simulink model "Dyn_PointMass_R2015B"  (R2015b)
settings: Solver=ode4  SolverMode=SingleTasking  StartTime=0.0  StopTime=simInit.TSIM  FixedStep=simInit.dt  MaxStep=simInit.dt  RelTol=1e-3
InitFcn:
  | close all
undefined symbols (not defined in the file): base_windspeed, constr, DE2019, DiscIntNeverNeededParam, ENVMT, Lbooth, loiterStates, params, simInit, T, winchParameter
libraries: simulink x40, simulink_extras x3, dspsigops x1
(part 4 of 5)

== matlab function Dyn_PointMass_R2015B/AirborneSystem/AeroAndPropForces/Aero_prop ==
  data: F_p_B output; airdata input; DE2019 parameter; delta_t input; F_a_B output; cl_w input; cd_w input; cl_e input; cd_e input; cl_r input; cd_r input; ENVMT parameter
% Copyright 2020 Delft University of Technology
%
% Licensed under the Apache License, Version 2.0 (the "License");
% you may not use this file except in compliance with the License.
% You may obtain a copy of the License at
%
%      http://www.apache.org/licenses/LICENSE-2.0
%
% Unless required by applicable law or agreed to in writing, software
% distributed under the License is distributed on an "AS IS" BASIS,
% WITHOUT WARRANTIES OR CONDITIONS OF ANY KIND, either express or implied.
% See the License for the specific language governing permissions and
% limitations under the License.

function [F_p_B,F_a_B] = simpleAero(airdata, DE2019, delta_t,cl_w,cd_w,cl_e,cd_e,cl_r,cd_r, ENVMT)
%simpleAero - Calculate aerodynamic and propulsive forces
%
% Syntax:  [F_p_B,F_a_B] = simpleAero(airdata, aircraft_struct, delta_t,cl_w,cd_w,cl_e,cd_e,cl_r,cd_r)
%
% Inputs:
%    airdata - Wind speed, angle of attack and side slip angle
%    DE2019 - Aircraft characteristics data structure
%    delta_t - Thrust force
%    cl_w - Lift coefficient wing
%    cd_w - Drag coefficient wing
%    cl_e - Lift coefficient elevator
%    cd_e - Drag coefficient elevator
%    cl_r - Lift coefficient rudder
%    cd_r - Drag coefficient rudder
%
% Outputs:
%    F_p_B  - Propulsive forces in body reference frame
%    F_a_B  - Total aircraft aerodynamic forces in body reference frame
%   
% Example: 
%    [F_p_B,F_a_B] = simpleAero(airdata, DE2019, delta_t,cl_w,cd_w,cl_e,cd_e,cl_r,cd_r)
%
% Other m-files required: none
% Subfunctions: none
% MAT-files required: none
%
% Author: Dylan Eijkelhof, M.Sc.
% Delft University of Technology
% email address: d.eijkelhof@tudelft.nl  
% December 2019; Last revision: 30-September-2019

%------------- BEGIN CODE --------------    
    F_a_B = zeros(3,1);
    F_p_B = zeros(3,1);

    Va = airdata(1);
    alpha = airdata(2);
    beta = airdata(3);    
    Vinf = [Va*cos(alpha)*cos(beta), Va*sin(beta), Va*sin(alpha)*cos(beta)];

    q = 0.5*ENVMT.rhos*Vinf(1)^2;
    
    %% Main Wing
    F_L_main = -cl_w*q*DE2019.S_ref;
    F_D_main = cd_w*q*DE2019.S_ref;
    
    F_x_mw = -F_D_main*cos(alpha) - F_L_main*sin(alpha);
    F_z_mw = F_L_main*cos(alpha);

    %% Elevator
    F_L_el = -cl_e*q*DE2019.S_el;
    F_D_el = -cd_e*q*DE2019.S_el;
    
    F_x_el = F_D_el*cos(alpha)*cos(beta) - F_L_el*sin(alpha)*cos(beta);
    F_z_el = F_L_el*cos(alpha);
   
    %% Rudder
    F_L_vs = 2*cl_r*q*DE2019.S_vs;
    F_D_vs = -2*cd_r*q*DE2019.S_vs;

    F_x_vs = F_D_vs*cos(alpha)*cos(beta);
    F_y_vs = -F_L_vs*cos(beta);
    
    %% Sum of forces
    F_a_B = [F_x_mw+F_x_el+F_x_vs;F_y_vs; F_z_mw+F_z_el];
    
    %% Motor
%     Vd = airdata(1) + delta_t * ( DE2019.k_motor - airdata(1) );
%     Fp_x = 0.5 * 1.225 * DE2019.S_prop * DE2019.C_prop * Vd * (Vd-airdata(1));
    %% No motor, direct feed through
    F_p_B = [delta_t;0;0];
%------------- END CODE -------------- 
end
%

== matlab function Dyn_PointMass_R2015B/AirborneSystem/FlightControlSystem/AirspeedController_SS_1/Airspeed_Brake/FeedforwardPart ==
  data: gamma input; BF output; nu_V input; ENVMT parameter; Drag_force input; DE2019 parameter
% Copyright 2021 Delft University of Technology
%
% Licensed under the Apache License, Version 2.0 (the "License");
% you may not use this file except in compliance with the License.
% You may obtain a copy of the License at
%
%      http://www.apache.org/licenses/LICENSE-2.0
%
% Unless required by applicable law or agreed to in writing, software
% distributed under the License is distributed on an "AS IS" BASIS,
% WITHOUT WARRANTIES OR CONDITIONS OF ANY KIND, either express or implied.
% See the License for the specific language governing permissions and
% limitations under the License.

function BF = feedforward_brake(gamma, nu_V,  ENVMT, Drag_force, DE2019)
%feedforward_brake - Brake force calculation for velocity decrease
%
% Inputs:
%    gamma      - Path angle (glideslope)
%    nu_V       - Controlled velocity parameter
%    ENVMT      - Environmental characteristics
%    Drag_force	- Drag
%    DE2019     - Aircraft characteristics
%
% Outputs:
%    BF          - Brake force
%
% Example: 
%    BF = feedforward_thrust(gamma, nu_V,  ENVMT, Drag_force, DE2019)
%
% Author: Sebastian Rapp, Ph.D., Revised by: Dylan Eijkelhof, M.Sc.
% Delft University of Technology
% email address: s.rapp@tudelft.nl
% email address: d.eijkelhof@tudelft.nl
% December 2019; Last revision: 06-October-2020

%-------------	BEGIN CODE	--------------

BF = DE2019.mass * ( ENVMT.g * sin(gamma) + nu_V ) + Drag_force; % required thrust

%-------------	 END CODE	--------------
end

== matlab function Dyn_PointMass_R2015B/AirborneSystem/FlightControlSystem/AirspeedController_SS_1/Airspeed_Brake/MATLAB Function ==
  data: F_a_B input; Drag output; AoA input
% Copyright 2021 Delft University of Technology
%
% Licensed under the Apache License, Version 2.0 (the "License");
% you may not use this file except in compliance with the License.
% You may obtain a copy of the License at
%
%      http://www.apache.org/licenses/LICENSE-2.0
%
% Unless required by applicable law or agreed to in writing, software
% distributed under the License is distributed on an "AS IS" BASIS,
% WITHOUT WARRANTIES OR CONDITIONS OF ANY KIND, either express or implied.
% See the License for the specific language governing permissions and
% limitations under the License.

function Drag  = estimate_drag(F_a_B, AoA)
%estimate_drag - Transform drag from B to A reference frame
%
% Inputs:
%    F_a_B     - Aerodynamic forces in body reference frame
%    AoA       - Angle of Attack
%
% Outputs:
%    Drag    - Drag force
%
% Example: 
%    [Drag] = estimate_drag(F_a_B, AoA)
%
% Author: Sebastian Rapp, Ph.D., Revised by: Dylan Eijkelhof, M.Sc.
% Delft University of Technology
% email address: s.rapp@tudelft.nl
% email address: d.eijkelhof@tudelft.nl
% December 2019; Last revision: 06-October-2020

%-------------	BEGIN CODE	--------------

F_a_A = [cos(AoA), 0, sin(AoA);
    0, 1, 0; 
    -sin(AoA), 0, cos(AoA)] * F_a_B;

Drag = -F_a_A(1);

%-------------	 END CODE	--------------

end

== matlab function Dyn_PointMass_R2015B/AirborneSystem/FlightControlSystem/AirspeedController_SS_1/Airspeed_Brake/hedging ==
  data: Drag_force input; gamma input; nu_V output; BF input; ENVMT parameter; DE2019 parameter
% Copyright 2021 Delft University of Technology
%
% Licensed under the Apache License, Version 2.0 (the "License");
% you may not use this file except in compliance with the License.
% You may obtain a copy of the License at
%
%      http://www.apache.org/licenses/LICENSE-2.0
%
% Unless required by applicable law or agreed to in writing, software
% distributed under the License is distributed on an "AS IS" BASIS,
% WITHOUT WARRANTIES OR CONDITIONS OF ANY KIND, either express or implied.
% See the License for the specific language governing permissions and
% limitations under the License.

function nu_V = hedgingV(Drag_force, gamma, BF, ENVMT, DE2019)

%hedgingV
%
% Inputs:
%    Drag_force	- Drag
%    gamma      - Path angle (glideslope)
%    BF         - Brake force
%    ENVMT      - Environmental characteristics
%    DE2019     - Aircraft characteristics
%
% Outputs:
%    nu_V       - Controlled velocity parameter
%
% Example: 
%    nu_V = hedgingV(Drag_force, gamma, BF, ENVMT, DE2019)
%
% Author: Sebastian Rapp, Ph.D., Revised by: Dylan Eijkelhof, M.Sc.
% Delft University of Technology
% email address: s.rapp@tudelft.nl
% email address: d.eijkelhof@tudelft.nl
% December 2019; Last revision: 06-October-2020

%-------------	BEGIN CODE	--------------

nu_V = (BF-Drag_force)/DE2019.mass - ENVMT.g * sin(gamma); 

%-------------	 END CODE	--------------
end

== matlab function Dyn_PointMass_R2015B/RequirementModelsAndLogging/MATLAB Function ==
  data: time input; eul input; stop_flag output; eul_old input
% Copyright 2021 Delft University of Technology
%
% Licensed under the Apache License, Version 2.0 (the "License");
% you may not use this file except in compliance with the License.
% You may obtain a copy of the License at
%
%      http://www.apache.org/licenses/LICENSE-2.0
%
% Unless required by applicable law or agreed to in writing, software
% distributed under the License is distributed on an "AS IS" BASIS,
% WITHOUT WARRANTIES OR CONDITIONS OF ANY KIND, either express or implied.
% See the License for the specific language governing permissions and
% limitations under the License.

function stop_flag = fcn(time, eul,eul_old)
phi = eul(1);
theta = eul(2);
% psi = eul(3);

phi_old = eul_old(1);
theta_old = eul_old(2);
% psi_old = eul_old(3);

if time>40
    if ((phi>pi/2 || phi<-pi/2) && sign(phi) ~= sign(phi_old))
        stop_flag = 1;
    elseif ((theta>pi/2 || theta<-pi/2) && sign(theta) ~= sign(theta_old))
        stop_flag = 1; 
%     elseif ((psi>pi/2 || psi<-pi/2) && sign(psi) ~= sign(psi_old))
%         stop_flag = 1; 
    else
        stop_flag = 0;
    end
else
    stop_flag = 0;
end
end

== matlab function Dyn_PointMass_R2015B/RequirementModelsAndLogging/MATLAB Function1 ==
  data: Lift output; F_a_B input; Drag output; AoA input
% Copyright 2021 Delft University of Technology
%
% Licensed under the Apache License, Version 2.0 (the "License");
% you may not use this file except in compliance with the License.
% You may obtain a copy of the License at
%
%      http://www.apache.org/licenses/LICENSE-2.0
%
% Unless required by applicable law or agreed to in writing, software
% distributed under the License is distributed on an "AS IS" BASIS,
% WITHOUT WARRANTIES OR CONDITIONS OF ANY KIND, either express or implied.
% See the License for the specific language governing permissions and
% limitations under the License.

function [Lift, Drag]  = estimate_drag(F_a_B, AoA)
%estimate_drag - Transform drag from B to A reference frame
%
% Inputs:
%    F_a_B     - Aerodynamic forces in body reference frame
%    AoA       - Angle of Attack
%
% Outputs:
%    Drag    - Drag force
%
% Example: 
%    [Drag] = estimate_drag(F_a_B, AoA)
%
% Author: Sebastian Rapp, Ph.D., Revised by: Dylan Eijkelhof, M.Sc.
% Delft University of Technology
% email address: s.rapp@tudelft.nl
% email address: d.eijkelhof@tudelft.nl
% December 2019; Last revision: 06-October-2020

%-------------	BEGIN CODE	--------------

F_a_A = [cos(AoA), 0, sin(AoA);
    0, 1, 0; 
    -sin(AoA), 0, cos(AoA)] * F_a_B;

Lift = -F_a_A(3);
Drag = -F_a_A(1);

%-------------	 END CODE	--------------

end

== matlab function Dyn_PointMass_R2015B/AirborneSystem/FlightControlSystem/PathFollowingController_SS_2/FlightOnFlatEarth (Retraction&Loitering)/CalculateAttitudeCmds/FlightPathLoopRetraction_Aerodynamic/FlightpathReferenceModels/SecondOrderReferenceModel_course/wrapto2pi ==
  data: u input; y output
% Copyright 2021 Delft University of Technology
%
% Licensed under the Apache License, Version 2.0 (the "License");
% you may not use this file except in compliance with the License.
% You may obtain a copy of the License at
%
%      http://www.apache.org/licenses/LICENSE-2.0
%
% Unless required by applicable law or agreed to in writing, software
% distributed under the License is distributed on an "AS IS" BASIS,
% WITHOUT WARRANTIES OR CONDITIONS OF ANY KIND, either express or implied.
% See the License for the specific language governing permissions and
% limitations under the License.

function y = wrap_to_2pi(u)
u = mod(u, 2*pi); 
if u > pi 
    du = mod(u,pi);
    y = -pi+du; 
elseif u < -pi 
    du = mod(u,-pi); 
    y = pi+du;
else
    y = u; 
end
end

== matlab function Dyn_PointMass_R2015B/Environment_SS_3/MATLAB Function1 ==
  data: v_w_u input; v_w_p_mat output
% Copyright 2021 Delft University of Technology
%
% Licensed under the Apache License, Version 2.0 (the "License");
% you may not use this file except in compliance with the License.
% You may obtain a copy of the License at
%
%      http://www.apache.org/licenses/LICENSE-2.0
%
% Unless required by applicable law or agreed to in writing, software
% distributed under the License is distributed on an "AS IS" BASIS,
% WITHOUT WARRANTIES OR CONDITIONS OF ANY KIND, either express or implied.
% See the License for the specific language governing permissions and
% limitations under the License.

function v_w_p_mat = fcn(v_w_u)

v_w_p_mat = zeros( 3, length( v_w_u) );
v_w_p_mat(1,:) = v_w_u';

== matlab function Dyn_PointMass_R2015B/AirborneSystem/FlightControlSystem/AirspeedController_SS_1/Airspeed_Control/FeedforwardPart ==
  data: gamma input; T output; nu_V input; ENVMT parameter; Drag_force input; DE2019 parameter
% Copyright 2021 Delft University of Technology
%
% Licensed under the Apache License, Version 2.0 (the "License");
% you may not use this file except in compliance with the License.
% You may obtain a copy of the License at
%
%      http://www.apache.org/licenses/LICENSE-2.0
%
% Unless required by applicable law or agreed to in writing, software
% distributed under the License is distributed on an "AS IS" BASIS,
% WITHOUT WARRANTIES OR CONDITIONS OF ANY KIND, either express or implied.
% See the License for the specific language governing permissions and
% limitations under the License.

function T = feedforward_thrust(gamma, nu_V,  ENVMT, Drag_force, DE2019)
%feedforward_thrust - Thrust calculation for velocity initialisation
%
% Inputs:
%    gamma      - Path angle (glideslope)
%    nu_V       - Controlled velocity parameter
%    ENVMT      - Environmental characteristics
%    Drag_force	- Drag
%    DE2019     - Aircraft characteristics
%
% Outputs:
%    T          - Thrust force
%
% Example: 
%    T = feedforward_thrust(gamma, nu_V,  ENVMT, Drag_force, DE2019)
%
% Author: Sebastian Rapp, Ph.D., Revised by: Dylan Eijkelhof, M.Sc.
% Delft University of Technology
% email address: s.rapp@tudelft.nl
% email address: d.eijkelhof@tudelft.nl
% December 2019; Last revision: 06-October-2020

%-------------	BEGIN CODE	--------------

T = DE2019.mass * ( ENVMT.g * sin(gamma) + nu_V ) + Drag_force; % required thrust

% Based on the quotient of commmanded to max. available thrust
% F_T_max = ENVMT.rhos * DE2019.S_prop * DE2019.C_prop * DE2019.k_motor * (DE2019.k_motor - Va);
% delta_t = T/F_T_max; 

%-------------	 END CODE	--------------
end

== stateflow chart Dyn_PointMass_R2015B/GroundSystem_SS_4/GroundControl/Select_init_sol_for_pathfollowing ==
  state Init
    entry: sol_init = x;
  state Pumping
    entry: sol_init = transition_phi;
  (default) -> Init
  Init -> Pumping : [fm == 6]
  data: x input; fm input; sol_init output; transition_phi input

== matlab function Dyn_PointMass_R2015B/AirborneSystem/FlightControlSystem/AirspeedController_SS_1/Airspeed_Control/MATLAB Function ==
  data: F_a_B input; Drag output; AoA input
% Copyright 2021 Delft University of Technology
%
% Licensed under the Apache License, Version 2.0 (the "License");
% you may not use this file except in compliance with the License.
% You may obtain a copy of the License at
%
%      http://www.apache.org/licenses/LICENSE-2.0
%
% Unless required by applicable law or agreed to in writing, software
% distributed under the License is distributed on an "AS IS" BASIS,
% WITHOUT WARRANTIES OR CONDITIONS OF ANY KIND, either express or implied.
% See the License for the specific language governing permissions and
% limitations under the License.

function Drag = estimate_drag(F_a_B, AoA)

%estimate_drag - Transform drag from B to A reference frame
%
% Inputs:
%    F_a_B     - Aerodynamic forces in body reference frame
%    AoA       - Angle of Attack
%
% Outputs:
%    Drag    - Drag force
%
% Example: 
%    Drag = estimate_drag(F_a_B, AoA)
%
% Author: Sebastian Rapp, Ph.D., Revised by: Dylan Eijkelhof, M.Sc.
% Delft University of Technology
% email address: s.rapp@tudelft.nl
% email address: d.eijkelhof@tudelft.nl
% December 2019; Last revision: 06-October-2020

%-------------	BEGIN CODE	--------------

F_a_A = [cos(AoA), 0, sin(AoA);
    0, 1, 0; 
    -sin(AoA), 0, cos(AoA)] * F_a_B;

Drag = -F_a_A(1);

%-------------	 END CODE	--------------
end

== matlab function Dyn_PointMass_R2015B/AirborneSystem/FlightControlSystem/AirspeedController_SS_1/Airspeed_Control/hedging ==
  data: Drag_force input; gamma input; nu_V output; T input; ENVMT parameter; DE2019 parameter
% Copyright 2021 Delft University of Technology
%
% Licensed under the Apache License, Version 2.0 (the "License");
% you may not use this file except in compliance with the License.
% You may obtain a copy of the License at
%
%      http://www.apache.org/licenses/LICENSE-2.0
%
% Unless required by applicable law or agreed to in writing, software
% distributed under the License is distributed on an "AS IS" BASIS,
% WITHOUT WARRANTIES OR CONDITIONS OF ANY KIND, either express or implied.
% See the License for the specific language governing permissions and
% limitations under the License.

function nu_V = hedgingV(Drag_force, gamma, T, ENVMT, DE2019)

%hedgingV
%
% Inputs:
%    Drag_force	- Drag
%    gamma      - Path angle (glideslope)
%    T          - Thrust force
%    ENVMT      - Environmental characteristics
%    DE2019     - Aircraft characteristics
%
% Outputs:
%    nu_V       - Controlled velocity parameter
%
% Example: 
%    nu_V = hedgingV(Drag_force, gamma, T, ENVMT, DE2019)
%
% Author: Sebastian Rapp, Ph.D., Revised by: Dylan Eijkelhof, M.Sc.
% Delft University of Technology
% email address: s.rapp@tudelft.nl
% email address: d.eijkelhof@tudelft.nl
% December 2019; Last revision: 06-October-2020

%-------------	BEGIN CODE	--------------

% Based on the quotient of commmanded to max. available thrust
% F_T_max = ENVMT.rhos * DE2019.S_prop * DE2019.C_prop * DE2019.k_motor * (DE2019.k_motor - Va);
% T = F_T_max * delta_t; 

nu_V = (T-Drag_force)/DE2019.mass - ENVMT.g * sin(gamma); 

%-------------	 END CODE	--------------
end

== stateflow chart Dyn_PointMass_R2015B/AirborneSystem/FlightControlSystem/AirspeedController_SS_1/Chart ==
  state Throttle_Off
    entry: throttle_on = 0;
  state Throttle_On
    entry: throttle_on = 1;
  (default) -> Throttle_Off
  Throttle_Off -> Throttle_On : [Va<Va_min || manual_switch_on || init_throttle_flag]
  Throttle_On -> Throttle_Off : [Va>Va_min+10&&manual_switch_on==0&& init_throttle_flag ==0]
  data: Va input; Va_min input; init_throttle_flag input; throttle_on output; manual_switch_on input

== stateflow chart Dyn_PointMass_R2015B/AirborneSystem/FlightControlSystem/AirspeedController_SS_1/Chart1 ==
  state Throttle_Off
    entry: brake_on = 0;
  state Throttle_On
    entry: brake_on = 1;
  (default) -> Throttle_Off
  Throttle_Off -> Throttle_On : [(manual_switch_on || brake_flag) && Ft <= Ft_retract+3000 && Vk>Vk_min]
  Throttle_On -> Throttle_Off : [(manual_switch_on==0&& brake_flag ==0) || Vk<Vk_min]
  data: brake_flag input; Vk input; brake_on output; manual_switch_on input; Ft input; Ft_retract parameter; Vk_min parameter

== matlab function Dyn_PointMass_R2015B/AirborneSystem/FlightControlSystem/AirspeedController_SS_1/MATLAB Function1 ==
  data: vel_k_O input; vel_k_h_W output; ENVMT parameter
% Copyright 2021 Delft University of Technology
%
% Licensed under the Apache License, Version 2.0 (the "License");
% you may not use this file except in compliance with the License.
% You may obtain a copy of the License at
%
%      http://www.apache.org/licenses/LICENSE-2.0
%
% Unless required by applicable law or agreed to in writing, software
% distributed under the License is distributed on an "AS IS" BASIS,
% WITHOUT WARRANTIES OR CONDITIONS OF ANY KIND, either express or implied.
% See the License for the specific language governing permissions and
% limitations under the License.

function vel_k_h_W    = fcn(vel_k_O,ENVMT)
%fcn - Calculate horizontal kinetic velocity in wind reference frame
%
% Inputs:
%    vel_k_O    - Kinetic velocity in inertial reference frame
%    ENVMT      - Environment characteristics
%
% Outputs:
%    vel_k_h_W  - Horizontal kinetic velocity magnitude in wind reference frame
%
%
% Author: Sebastian Rapp, Ph.D., Revised by: Dylan Eijkelhof, M.Sc.
% Delft University of Technology
% email address: s.rapp@tudelft.nl
% email address: d.eijkelhof@tudelft.nl
% December 2019; Last revision: 06-October-2020

%-------------	BEGIN CODE	--------------

vel_k_W = transformFromOtoW(ENVMT.windDirection_rad, vel_k_O);

vel_k_h_W = sign(-vel_k_W(1))*sqrt( vel_k_W(1)^2 + vel_k_W(2)^2 );

%-------------	 END CODE	--------------
end

== stateflow chart Dyn_PointMass_R2015B/GroundSystem_SS_4/StateMachine/StateMachine ==
  state loiter
    entry: flightMode = 1;
    during: F_t_set = Ft_set_loiter;
    entry: init_throttle_flag = 1;
    entry: sub_flight_state = 1;
  state Traction4 % slowly increase tether force
    entry: flightMode=5;
    during: F_t_set = calcSetpoint(alpha2,Ft_set_prev,Ft_set_loiter);
    exit: init_throttle_flag = 1;
    entry: sub_flight_state = 2;
  note: F_t_m>F_set_retraction
  note: pos_x_W<x_trigger_transition
  state Retraction3 [commented out]
    entry: flightMode=6;
    entry: F_t_set =calcSetpoint(1,Ft_set_prev,3000);
    %entry: F_t_set = 0;
    entry: reelin_flag = 1;
    entry: sub_flight_state = 8;
    entry: path_captured_flag = 0;
  state Traction2 % slowly increase tether force
    entry: flightMode=5;
    during: F_t_set = calcSetpoint(alpha2,Ft_set_prev,F_T_traction_set);
    exit: init_throttle_flag = 1;
    entry: sub_flight_state = 2;
  state Retraction1
    entry: flightMode=6;
    entry: F_t_set =calcSetpoint(alpha2,F_set_retraction,Ft_set_prev);
    entry: reelin_flag = 1;
    entry: sub_flight_state = 7;
    entry: path_captured_flag = 0;
  state Retraction
    entry: flightMode=6;
    entry: reelin_flag = 1;
    during: F_t_set = calcSetpoint(alpha2,F_set_retraction,Ft_set_prev);
    entry: sub_flight_state = 6;
  state Traction1
    entry: flightMode=5;
    during: F_t_set = calcSetpoint(alpha2,Ft_set_prev,F_T_traction_set);
    entry: sub_flight_state = 3;
  state Traction3
    entry: flightMode=5;
    entry: path_captured_flag = 1;
    entry: init_throttle_flag = 0;
    during: F_t_set = calcSetpoint(alpha2,Ft_set_prev,F_T_traction_set);
    entry: sub_flight_state = 4;
  state Trans2Retract
    entry: flightMode=5;
    during: F_t_set = calcSetpoint(alpha2,Ft_set_prev,F_T_traction_set);
    entry: sub_flight_state = 5;
  (default) -> loiter
  loiter -> Traction4 % slowly increase tether force : [trigger_kite_mode == 1]
  Traction4 % slowly increase tether force -> Traction2 % slowly increase tether force : [pre_pc_mode_flag==0]
  Retraction1 -> Retraction3 [commented out] : [x_trigger_transition>0]
  Retraction1 -> Traction1 : [pos_x_W<x_trigger_transition]
  Traction2 % slowly increase tether force -> Traction3 : [long_kite>0]
  Retraction -> Retraction1 : [F_t_m<1.1*F_set_retraction]
  (junction 286) -> Retraction
  Traction1 -> Traction3 : [cross_track_error < crosstrackerror_condition&&Va>=Vamin]
  Traction3 -> Trans2Retract : [(l_t>l_t_max||init_retraction_flag)]
  Traction3 -> Trans2Retract [commented out] : [(l_t>l_t_max||init_retraction_flag)&& (path_parameter_s >= (5*pi/3+.5*pi/180) && path_parameter_s <=5*pi/3+1*pi/180)]
  Traction3 -> Trans2Retract [commented out] : [(l_t>l_t_max||init_retraction_flag)&& (path_parameter_s >= (2*pi/3+.5*pi/180) && path_parameter_s <= 2*pi/3+1*pi/180)]
  Trans2Retract -> (junction 286) [order 1] : [path_parameter_s >= (pi/2+.5*pi/180) && path_parameter_s <= pi/2+1*pi/180]
  (junction 319) -> (junction 286)
  Trans2Retract -> (junction 319) [order 2] : [path_parameter_s >= (3*pi/2+.5*pi/180) && path_parameter_s <=3*pi/2+1*pi/180]
  (junction 348) -> (junction 319) [commented out]
  Trans2Retract -> (junction 348) [commented out] : [Chi >= (0-0.5*pi/180) && Chi <= 0+0.5*pi/180]
  data: Ft_set function_output; alpha1_ function_input; Ft_set_prev_ function_input; F_T_traction_set_ function_input; flightMode output; long_kite input; lat_kite input; l_t input; F_t input; Lbooth parameter; pos_x_W input; pos_y_W input; F_t_set output; F_T_traction_set parameter double; F_set_retraction parameter; a_booth parameter; b_booth parameter; l_t_min parameter; lat_trans parameter; l_t_max parameter; Ft_set_prev input; alpha2 parameter; Va input; lat_init input; traction_trigger input; cross_track_error input; trigger_kite_mode input; init_throttle_flag output size=1; crosstrackerror_condition parameter; Vamin parameter; init_retraction_flag input; Ft_set_loiter parameter; phi0 input; F_t_m input; sub_flight_state output =1; pre_pc_mode_flag input; path_parameter_s input; sim_time input; reelin_flag local; path_captured_flag local; x_trigger_transition input; side local; Chi input
  function Ft_set = calcSetpoint(alpha1_,Ft_set_prev_, F_T_traction_set_):
    | % Copyright 2020 Delft University of Technology
    | %
    | % Licensed under the Apache License, Version 2.0 (the "License");
    | % you may not use this file except in compliance with the License.
    | % You may obtain a copy of the License at
    | %
    | %      http://www.apache.org/licenses/LICENSE-2.0
    | %
    | % Unless required by applicable law or agreed to in writing, software
    | % distributed under the License is distributed on an "AS IS" BASIS,
    | % WITHOUT WARRANTIES OR CONDITIONS OF ANY KIND, either express or implied.
    | % See the License for the specific language governing permissions and
    | % limitations under the License. 
    | 
    | function Ft_set = calcSetpoint(alpha1_,Ft_set_prev_, F_T_traction_set_)
    |  
    | Ft_set =  alpha1_ * F_T_traction_set_ +(1-alpha1_)*Ft_set_prev_;
    | 
    | end

== matlab function Dyn_PointMass_R2015B/AirborneSystem/FlightControlSystem/PathFollowingController_SS_2/FlightOnFlatEarth (Retraction&Loitering)/CalculateAttitudeCmds/FlightPathLoopRetraction_Aerodynamic/PIController_opt/wrapCourse ==
  data: chi_ref input; e_course output; chi input
% Copyright 2021 Delft University of Technology
%
% Licensed under the Apache License, Version 2.0 (the "License");
% you may not use this file except in compliance with the License.
% You may obtain a copy of the License at
%
%      http://www.apache.org/licenses/LICENSE-2.0
%
% Unless required by applicable law or agreed to in writing, software
% distributed under the License is distributed on an "AS IS" BASIS,
% WITHOUT WARRANTIES OR CONDITIONS OF ANY KIND, either express or implied.
% See the License for the specific language governing permissions and
% limitations under the License.

function e_course = course_error(chi_ref, chi)
%course_error - Calculate the error between commanded and actual course angle
%
% Inputs:
%    chi_ref  - Required chi
%    chi      - Actual chi
%
% Outputs:
%    e_course - Course (heading) error
%
% Author: Sebastian Rapp, Ph.D., Revised by: Dylan Eijkelhof, M.Sc.
% Delft University of Technology
% email address: s.rapp@tudelft.nl
% email address: d.eijkelhof@tudelft.nl
% December 2019; Last revision: 06-October-2020

%-------------	BEGIN CODE	--------------

%#codegen
% The vectors are lying in the tangential plane attached to the current
% position on the small earth.
p_bearing_vec =   [cos(chi);         sin(chi);         0];
p_bearing_vec = p_bearing_vec/norm(p_bearing_vec); 
ref_bearing_vec = [cos(chi_ref); sin(chi_ref); 0];
ref_bearing_vec = ref_bearing_vec/norm(ref_bearing_vec); 

e_z = cross( ref_bearing_vec, p_bearing_vec ); 

dot_product = dot( ref_bearing_vec, p_bearing_vec ); 
if dot_product > 1 
    dot_product = 1; 
end
if dot_product < -1 
    dot_product = -1; 
end

e_course = - sign( e_z(3) ) * acos( dot_product );
%-------------	 END CODE	--------------
end

== matlab function Dyn_PointMass_R2015B/Visualisation/Visualisation ==
  settings: updateMethod=DISCRETE  sampleTime=sample_time_vis
  data: t input; p_t_x input; p_t_y input; p_t_z input; phi0_update input; pos_O input; eta_OB input; params parameter; ENVMT parameter; sub_flight_state input; arcP input; sampletime input
% Copyright 2021 Delft University of Technology
%
% Licensed under the Apache License, Version 2.0 (the "License");
% you may not use this file except in compliance with the License.
% You may obtain a copy of the License at
%
%      http://www.apache.org/licenses/LICENSE-2.0
%
% Unless required by applicable law or agreed to in writing, software
% distributed under the License is distributed on an "AS IS" BASIS,
% WITHOUT WARRANTIES OR CONDITIONS OF ANY KIND, either express or implied.
% See the License for the specific language governing permissions and
% limitations under the License.

function Visualisation(t,p_t_x,p_t_y,p_t_z,phi0_update, pos_O,eta_OB,params, ENVMT, sub_flight_state, arcP, sampletime)   
    persistent handleTether
    persistent pathpoints
    persistent referencePath
    persistent Vert
    persistent handlePlane
    persistent retractionPath
    
    coder.extrinsic('plot3','patch','animatedline','addpoints');
 
    %% Figure settings
    if t==0
        figure(99)
%         addToolbarExplorationButtons(gcf)
        xlabel('x_W (m)');%, 'interpreter', 'latex')
        ylabel('y_W (m)');%, 'interpreter', 'latex')
        zlabel('z_W (m)');%, 'interpreter', 'latex')

        grid on
        box on;
        axis equal; hold on;

        view(30,21); % set the vieew angle for figure

        ax = [-500 1500];
        ay = [-1000 1000];
        az = [0 1200];
        axis([ax,ay,az]);  hold on

        X = [ax(1);ax(2);ax(2);ax(1)];
        Y = [ay(1);ay(1);ay(2);ay(2)];
        Z = [0;0;0;0];

        c = [0 1 0; % red
        0 1 0; % green
        0 1 0;
        0 1 0];
        fill3(X,Y,Z, c(:,2),'EdgeColor','none','FaceColor',c(1,:),'FaceAlpha',0.1);
    end
    
    %% Draw tether particles
    if isempty(handleTether)
 
        M_WO = [cos(ENVMT.windDirection_rad), sin(ENVMT.windDirection_rad), 0;
        sin(ENVMT.windDirection_rad), -cos(ENVMT.windDirection_rad), 0;
        0, 0, -1];
        pos_W = M_WO*[pos_O(1);pos_O(2);pos_O(3)];
        handleTether = plot3( [0;flipud(p_t_x);pos_W(1)], [0;flipud(p_t_y);pos_W(2)],[0;flipud(p_t_z);pos_W(3)],...
            '-', 'color', [0.1 0.1 0.1], 'Markersize',2, 'Linewidth', 1.2,...
            'MarkerFaceColor', [0.3 0.3 0.3]); hold on;
    end
    
    %% Draw aircraft
    if isempty(handlePlane)
        pn = pos_O(1);
        pe = pos_O(2);
        pd = pos_O(3);
        phi = eta_OB(1);
        theta = eta_OB(2);
        psi = eta_OB(3);
        
        M_WO = [cos(ENVMT.windDirection_rad), sin(ENVMT.windDirection_rad), 0;
        sin(ENVMT.windDirection_rad), -cos(ENVMT.windDirection_rad), 0;
        0, 0, -1];
        
        scale = 6;
%         [F, Vert, C] = rndread('plane_thesis_big.stl');
        Image_kite = coder.load('plane_image.mat','F','Verti','C');
        F = Image_kite.F;
        Verti = Image_kite.Verti;
        C = Image_kite.C;
        Vert = scale*Verti'; 
        V = [ cos(psi)*cos(theta) , cos(psi)*sin(phi)*sin(theta) - cos(phi)*sin(psi) , sin(phi)*sin(psi) + cos(phi)*cos(psi)*sin(theta);
            cos(theta)*sin(psi)   , cos(phi)*cos(psi) + sin(phi)*sin(psi)*sin(theta) , cos(phi)*sin(psi)*sin(theta) - cos(psi)*sin(phi);
               -sin(theta)        ,             cos(theta)*sin(phi)                  ,             cos(phi)*cos(theta)                 ]...
               * Vert;
        V = V + [pn*ones(1,size(V,2));pe*ones(1,size(V,2));pd*ones(1,size(V,2))];
        V = M_WO*V;
        col =  [ 57/255, 106/255, 177/255  ];
        handlePlane = patch('faces', F, 'vertices' ,V');
        set(handlePlane, 'facec', 'b');              % Set the face color (force it)
        set(handlePlane, 'FaceVertexCData', C);       % Set the color (from file)
        set(handlePlane, 'EdgeColor','none');
        set(handlePlane, 'FaceLighting', 'none');
        set(handlePlane, 'FaceColor', col );
    end
    
    %% Draw black thin trail behind kite
    if isempty(pathpoints)
        pathpoints = animatedline('Linestyle','-','color', [85/255, 85/255, 85/255 ], 'Linewidth', .5);
    end
    
    %% Draw red target figure of 8 (traction)
    if isempty(referencePath)
        
        Lbooth.a = params.a_booth*params.b_booth;
        Lbooth.b = params.b_booth;
        Lbooth.phi0 = phi0_update;
        
        s = 0 : 0.01 : 2*pi;
        l_tether = norm(pos_O);
        Lem.a = Lbooth.a/(l_tether); 
        Lem.b = Lbooth.b/(l_tether); 
        Lem.phi0 = Lbooth.phi0;
        long_P = Lem.b * sin(s) ./( 1+(Lem.a/Lem.b*cos(s)).^2 );
        lat_P =   Lem.a * sin(s).*cos(s) ./ ( 1+(Lem.a/Lem.b*cos(s)).^2 );
        p_P = [ cos(long_P).*cos(lat_P);sin(long_P).*cos(lat_P);sin(lat_P)]*l_tether;
        phi_p_mean = Lbooth.phi0;
        M_WP = [cos(phi_p_mean),0, -sin(phi_p_mean);0, 1, 0;  sin(phi_p_mean),0, cos(phi_p_mean)];
        p_W = M_WP * p_P;
        referencePath = plot3( p_W(1,:),p_W(2,:),p_W(3,:) , '-', 'color', [1 0.3 0.3],'Linewidth', 1.5);
    end
    
    %% Draw red retraction path (retraction)
    if isempty(retractionPath)
        retractionPath = plot3( arcP(1,:),arcP(2,:),arcP(3,:), '--', 'color', [1 0.3 0.3],'Linewidth', .5);
    end
    
    if (mod(t,sampletime)==0 && t~=0)
        %% Change each element on figure to current positions
        Lbooth.a = params.a_booth*params.b_booth;
        Lbooth.b = params.b_booth;
        Lbooth.phi0 = phi0_update;
        
        pn = pos_O(1);
        pe = pos_O(2);
        pd = pos_O(3);
        phi = eta_OB(1);
        theta = eta_OB(2);
        psi = eta_OB(3);
        
        M_WO = [cos(ENVMT.windDirection_rad), sin(ENVMT.windDirection_rad), 0;
        sin(ENVMT.windDirection_rad), -cos(ENVMT.windDirection_rad), 0;
        0, 0, -1];
        
        % Tether
        set(handleTether,'XData',[0;flipud(p_t_x);-pn], 'YData',[0;flipud(p_t_y);pe],'ZData',[0;flipud(p_t_z);-pd]);
        
        % Kite
        V = [ cos(psi)*cos(theta), cos(psi)*sin(phi)*sin(theta) - cos(phi)*sin(psi), sin(phi)*sin(psi) + cos(phi)*cos(psi)*sin(theta);
            cos(theta)*sin(psi), cos(phi)*cos(psi) + sin(phi)*sin(psi)*sin(theta), cos(phi)*sin(psi)*sin(theta) - cos(psi)*sin(phi);
            -sin(theta),                              cos(theta)*sin(phi),                              cos(phi)*cos(theta)] * Vert;
        V = V + [pn*ones(1,size(V,2));pe*ones(1,size(V,2));pd*ones(1,size(V,2))];
        V = M_WO*V;
        set(handlePlane, 'Vertices', V');
        
        % Trail
        pos_W = M_WO*[pn;pe;pd];
        addpoints(pathpoints,pos_W(1), pos_W(2),pos_W(3))
        
        % Target figure (traction)
        s = 0 : 0.01 : 2*pi;
        l_tether = norm(pos_O);
        Lem.a = Lbooth.a/(l_tether); 
        Lem.b = Lbooth.b/(l_tether); 
        Lem.phi0 = Lbooth.phi0;
        long_P = Lem.b * sin(s) ./( 1+(Lem.a/Lem.b*cos(s)).^2 );
        lat_P =   Lem.a * sin(s).*cos(s) ./ ( 1+(Lem.a/Lem.b*cos(s)).^2 );
        p_P = [ cos(long_P).*cos(lat_P);sin(long_P).*cos(lat_P);sin(lat_P)]*l_tether;
        phi_p_mean = Lbooth.phi0;
        M_WP = [cos(phi_p_mean),0, -sin(phi_p_mean);0, 1, 0;  sin(phi_p_mean),0, cos(phi_p_mean)];
        p_W = M_WP * p_P;
        set(referencePath,'XData',p_W(1,:),'YData',p_W(2,:),'ZData',p_W(3,:));
        
        % Target path (retraction)
        if sub_flight_state >= 6
            set(retractionPath,'XData',arcP(1,:),'YData',arcP(2,:),'ZData',arcP(3,:));
        else
            set(retractionPath,'XData',zeros(1,size(arcP,2)),'YData',zeros(1,size(arcP,2)),'ZData',zeros(1,size(arcP,2)));
        end
    end

== matlab function Dyn_PointMass_R2015B/AirborneSystem/FlightControlSystem/PathFollowingController_SS_2/FlightOnFlatEarth (Retraction&Loitering)/CalculateAttitudeCmds/FlightPathLoopRetraction_Aerodynamic/TrafoPathKin2PathAero ==
  data: Va input; beta input; Vg input; v_w_O input; chi_k input; gamma_k input; chi_a output; gamma_a output
% Copyright 2021 Delft University of Technology
%
% Licensed under the Apache License, Version 2.0 (the "License");
% you may not use this file except in compliance with the License.
% You may obtain a copy of the License at
%
%      http://www.apache.org/licenses/LICENSE-2.0
%
% Unless required by applicable law or agreed to in writing, software
% distributed under the License is distributed on an "AS IS" BASIS,
% WITHOUT WARRANTIES OR CONDITIONS OF ANY KIND, either express or implied.
% See the License for the specific language governing permissions and
% limitations under the License.

function [chi_a, gamma_a] = PathKin2PathAero(Va, beta, Vg, v_w_O, chi_k, gamma_k)
%PathKin2PathAero - transform kinetic path angles into aerodynamic path
%                   angles
%
% Inputs:
%    Va         - Aircraft velocity component on body x axis
%    beta       - Aircraft side slip angle
%    Vg         - Kinetic velocity magnitude
%    v_w_O      - Wind velocity at aircraft in inertial reference frame
%    chi_k      - Kinetic course heading
%    gamma_k    - Kinetic path angle
%
% Outputs:
%    chi_a      - Aerodynamic course heading
%    gamma_a 	- Aerodynamic path angle
%
% Example: [chi_a, gamma_a] = fcn(Va, beta, Vg, v_w_O, chi_k, gamma_k)
%
% Other m-files required: none
% Subfunctions: none
% MAT-files required: none
%
% Author: Sebastian Rapp, Phd.
% Delft University of Technology
% email address: s.rapp@tudelft.nl  

%------------- BEGIN CODE --------------
gamma_a = asin( max( min( (Vg*sin(gamma_k)+v_w_O(3))/(Va+1e-9),1), -1) );
chi_a = beta + chi_k - asin( max( min( 1/(Va*cos(gamma_a)) * (v_w_O(1)*(-sin(chi_k))+v_w_O(2)*cos(chi_k)),1), -1) );
%------------- END CODE --------------
end

== stateflow chart Dyn_PointMass_R2015B/AirborneSystem/FlightControlSystem/PathFollowingController_SS_2/FlightOnFlatEarth (Retraction&Loitering)/GuidanceFlatEarth/LoiteringGuidance/Loiter ==
  state initLoiter
    during: [e_track,course_des,valid_transition_region_flag]  = initLoiterGuidance(kp_course_init, p_x_W,p_y_W, pos_OLoiter_W, R_init_loiter, windDir, Vk, validTransReg_start, validTransReg_end);
  (default) -> (junction 217)
  (junction 217) -> initLoiter : [1]
  data: delta function_output; kp_ function_input; p_x_W_ function_input; p_y_W_ function_input; pos_OLoiter_W_ function_input; R_ function_input; windDirection_rad_ function_input; Vk_ function_input; course_des_ function_output; valid_transition_region_flag_ function_output; validTransReg_start_ function_input; validTransReg_end_ function_input; course_des output; p_y_W input; course_k input; p_x_W input; Vk input; kp_course_init parameter; validTransReg_start parameter; validTransReg_end parameter; pos_OLoiter_W parameter; R_init_loiter parameter; valid_transition_region_flag output; e_track output; reset_flag input; windDir input
  function [delta, course_des_,valid_transition_region_flag_]  = initLoiterGuidance(kp_, p_x_W_,p_y_W_, pos_OLoiter_W_, R_, windDirection_rad_, Vk_, validTransReg_start_, validTransReg_end_):
    | % Copyright 2020 Delft University of Technology
    | %
    | % Licensed under the Apache License, Version 2.0 (the "License");
    | % you may not use this file except in compliance with the License.
    | % You may obtain a copy of the License at
    | %
    | %      http://www.apache.org/licenses/LICENSE-2.0
    | %
    | % Unless required by applicable law or agreed to in writing, software
    | % distributed under the License is distributed on an "AS IS" BASIS,
    | % WITHOUT WARRANTIES OR CONDITIONS OF ANY KIND, either express or implied.
    | % See the License for the specific language governing permissions and
    | % limitations under the License. 
    | 
    | function [delta, course_des_,valid_transition_region_flag_]  = initLoiterGuidance(kp_, p_x_W_,p_y_W_, pos_OLoiter_W_, R_, windDirection_rad_, Vk_, validTransReg_start_, validTransReg_end_) 
    | 
    | %#codegen
    | 
    | %% LOITER GUIDANCE: compare with approach where height and ground track is controlled independently
    | p_W_ = [p_x_W_; p_y_W_; 0];
    | 
    | pos_OLoiter_W_(3) = 0;
    | r_circ_W =  pos_OLoiter_W_;
    | 
    | 
    | p_P =  ( p_W_ - r_circ_W );
    | V = [1, 0; 0, 1; 0, 0];
    | p_P = V*((V'*V)\eye(2))*V'*p_P;
    | p_P = p_P / norm(p_P) * R_;
    | 
    | s_star = atan2( p_P(2), p_P(1) );
    | t_P = [-sin(s_star); cos(s_star); 0]*R_;
    | t_W = t_P;% + r_circ_W;
    | t_O = transformFromWtoO(windDirection_rad_, t_W);
    | 
    | p_proj_W =  p_P + r_circ_W;
    | delta_W = p_W_ - p_proj_W;
    | delta = norm( delta_W );
    | 
    | 
    | epx = t_W/norm(t_W);
    | epy = delta_W/norm(delta_W);
    | epz = cross( epx, epy ); epz = epz/norm(epz);
    | 
    | chi_star = atan2(t_O(2), t_O(1));
    | deltaChi = sign(epz(3))*asin( max( min( delta*kp_/Vk_ ,1),-1) );  %atan2( delta, 0.1*R_ );
    | 
    | course_des_ = chi_star + deltaChi;
    | 
    | bearing_O = [cos(course_des_); sin(course_des_); 0];
    | bearing_W = transformFromOtoW(windDirection_rad_, bearing_O);
    | 
    | if s_star > validTransReg_start_ && s_star < validTransReg_end_
    |     valid_transition_region_flag_ = 1;
    | else
    |     valid_transition_region_flag_ = 0;
    | end

== matlab function Dyn_PointMass_R2015B/AirborneSystem/FlightControlSystem/PathFollowingController_SS_2/FlightOnFlatEarth (Retraction&Loitering)/GuidanceFlatEarth/Retraction_Nav/MATLAB Function1 ==
  data: vel_k_O input; vel_k_h_W output; ENVMT parameter
% Copyright 2021 Delft University of Technology
%
% Licensed under the Apache License, Version 2.0 (the "License");
% you may not use this file except in compliance with the License.
% You may obtain a copy of the License at
%
%      http://www.apache.org/licenses/LICENSE-2.0
%
% Unless required by applicable law or agreed to in writing, software
% distributed under the License is distributed on an "AS IS" BASIS,
% WITHOUT WARRANTIES OR CONDITIONS OF ANY KIND, either express or implied.
% See the License for the specific language governing permissions and
% limitations under the License.

function vel_k_h_W    = fcn(vel_k_O,ENVMT)
%fcn - Calculate horizontal kinetic velocity in wind reference frame
%
% Inputs:
%    vel_k_O    - Kinetic velocity in inertial reference frame
%    ENVMT      - Environment characteristics
%
% Outputs:
%    vel_k_h_W  - Horizontal kinetic velocity magnitude in wind reference frame
%
%
% Author: Sebastian Rapp, Ph.D., Revised by: Dylan Eijkelhof, M.Sc.
% Delft University of Technology
% email address: s.rapp@tudelft.nl
% email address: d.eijkelhof@tudelft.nl
% December 2019; Last revision: 06-October-2020

%-------------	BEGIN CODE	--------------

vel_k_W = transformFromOtoW(ENVMT.windDirection_rad, vel_k_O);

vel_k_h_W = sqrt( vel_k_W(1)^2 + vel_k_W(2)^2 );

%-------------	 END CODE	--------------
end
